simulink model "ReadHectorSlam_Model"  (R2023a)
settings: Solver=FixedStepAuto  StartTime=0.0  StopTime=Inf  RelTol=1e-3
model workspace (MAT data in the model file):
  SL_ROS_VariableLengthArrays_MaxSizes.CommonInfo.ArrayTruncateAction = 'EmitWarning'
  SL_ROS_VariableLengthArrays_MaxSizes.MsgTypeMap = containers.Map
  SL_ROS_VariableLengthArrays_MaxSizes.MsgTypeMap.serialization.keys = {'nav_msgs/OccupancyGrid'}
  SL_ROS_VariableLengthArrays_MaxSizes.MsgTypeMap.serialization.values{1}.PropertyName = 'Data'
  SL_ROS_VariableLengthArrays_MaxSizes.MsgTypeMap.serialization.values{1}.DataType = 'int8'
  SL_ROS_VariableLengthArrays_MaxSizes.MsgTypeMap.serialization.values{1}.MaxLength = 128
  SL_ROS_VariableLengthArrays_MaxSizes.MsgTypeMap.serialization.uniformity = 0
  SL_ROS_VariableLengthArrays_MaxSizes.MsgTypeMap.serialization.keyType = 'char'
  SL_ROS_VariableLengthArrays_MaxSizes.MsgTypeMap.serialization.valueType = 'any'
values from neighbouring files (symbols this model uses):
  map = occupancyMap(cMap,20)    [FrontierPractice.m]    (also in LidarSlam_interp.m = buildMap(scans, poses, obj.mapResolution, obj.maxLidarRange); ReadHectorSlam.m = readOccupancyGrid(mapMsg))
libraries: robotlib x1
settings Model: Creator=cesf9  LastModifiedBy=cesf9
settings OptimizationCC: EnhancedBackFolding=on  PassReuseOutputArgsAs=Individual arguments  ZeroExternalMemoryAtStartup=off  ZeroInternalMemoryAtStartup=off  MaxStackSize=64  OptimizeBlockOrder=speed  DifferentSizesBufferReuse=on  OptimizationCustomize=off  EfficientTunableParamExpr=on
settings DebuggingCC: ParameterTunabilityLossMsg=error
settings HardwareCC: ProdBitPerPointer=32  ProdBitPerSizeT=32  ProdBitPerPtrDiffT=32  ProdLargestAtomicFloat=None  ProdIntDivRoundTo=Undefined  ProdEndianess=Unspecified  ProdWordSize=32  ProdHWDeviceType=Generic->Unspecified (assume 32-bit Generic)  UseEmbeddedCoderFeatures=off
settings SFSimCC: MATLABDynamicMemAlloc=off
settings RTWCC: Description=Embedded Coder  SystemTargetFile=ert.tlc  HardwareBoard=Robot Operating System (ROS)  TLCOptions="-aInlineSetEventsForThisBaseRateFcn=TLC_FALSE -aSuppressMultiTaskScheduler=TLC_FALSE  -aRateBasedStepFcn=0"  TemplateMakefile=ert_default_tmf  Toolchain=Catkin  TargetLang=C++
settings CodeAppCC: ForceParamTrailComments=on  IgnoreCustomStorageClasses=off  OperatorAnnotations=on  SimulinkDataObjDesc=on  SFDataObjDesc=on  InsertBlockDesc=on
settings ERTTargetCC: SupportNonInlinedSFcns=on

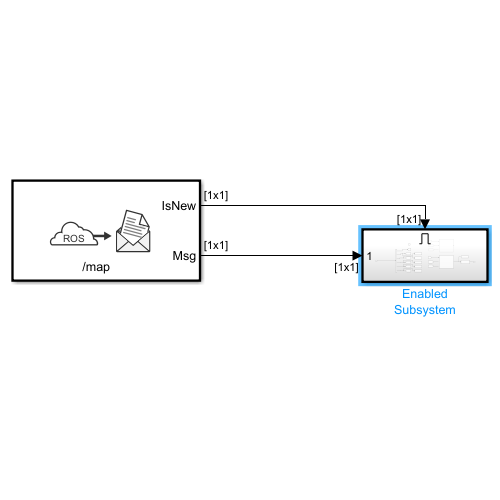
[thumbnail: Simulink's stored preview of the top-level diagram]
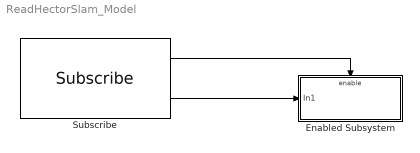
== system ReadHectorSlam_Model ==
  Enabled Subsystem : Subsystem  TreatAsAtomicUnit=on
  Subscribe : robotlib/Subscribe  topicSource=Select from ROS network  topic=/map  messageType=nav_msgs/OccupancyGrid  SampleTime=-1  legacyBusStruct=off  messageQueueLength=1
  wires:
  Subscribe/1 -> Enabled Subsystem/Enable
  Subscribe/2 -> Enabled Subsystem/1(In1)

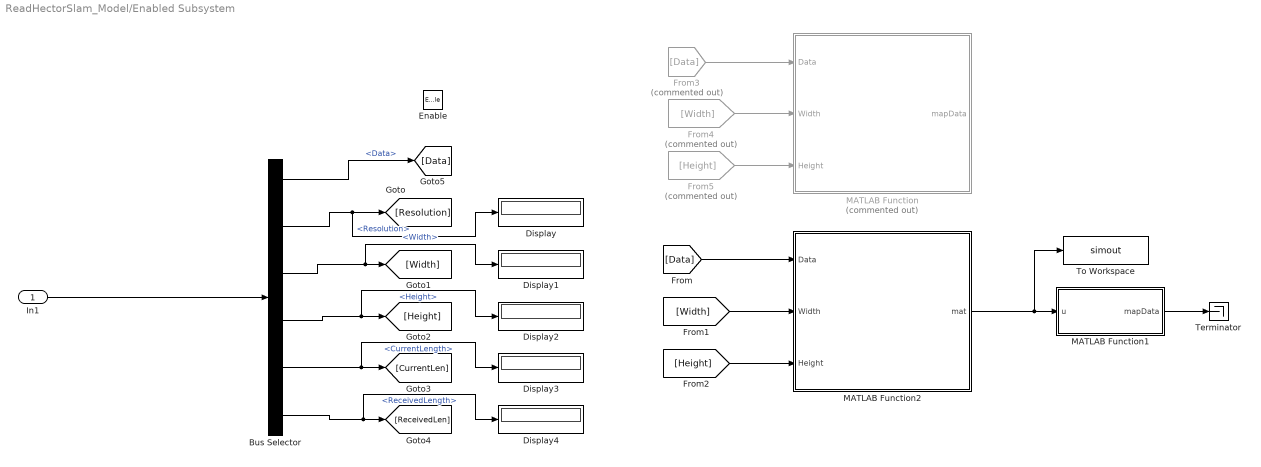
== system ReadHectorSlam_Model/Enabled Subsystem ==
  In1 : Inport
  Enable : EnablePort
  Bus Selector : BusSelector  OutputSignals=Data,Info.Resolution,Info.Width,Info.Height,Data_SL_Info.CurrentLength,Data_SL_Info.ReceivedLength
  Display{,1..4} (5 alike) : Display
  From3 : From  Commented=on  GotoTag=Data
  From4 : From  Commented=on  GotoTag=Width
  From5 : From  Commented=on  GotoTag=Height
  MATLAB Function : MATLAB Function  Commented=on  TreatAsAtomicUnit=on
  MATLAB Function1 : MATLAB Function  TreatAsAtomicUnit=on
  MATLAB Function2 : Subsystem
      mask help: Simulink:masks:GenSFuncDesc_MD
      mask Help: eval('feval(''rtwprivate'',''rtwhelpview'',''rtw_sfcn_block'')');
  Terminator : Terminator
  To Workspace : ToWorkspace  VariableName=simout  SaveFormat=Structure With Time  SampleTime=-1
  wires:
  In1/1 -> Bus Selector/1
  Bus Selector/2 -> Display/1, [Resolution]  "<Resolution>"
  Bus Selector/3 -> Display1/1, [Width]  "<Width>"
  Bus Selector/4 -> Display2/1, [Height]  "<Height>"
  Bus Selector/5 -> Display3/1, [CurrentLen]  "<CurrentLength>"
  Bus Selector/6 -> Display4/1, [ReceivedLen]  "<ReceivedLength>"
  Bus Selector/1 -> [Data]  "<Data>"
  [Data] -> MATLAB Function2/1(Data)
  [Width] -> MATLAB Function2/2(Width)
  [Height] -> MATLAB Function2/3(Height)
  MATLAB Function2/1(mat) -> To Workspace/1, MATLAB Function1/1(u)
  From4/1 -> MATLAB Function/2(Width)
  From3/1 -> MATLAB Function/1(Data)
  From5/1 -> MATLAB Function/3(Height)
  MATLAB Function1/1(mapData) -> Terminator/1

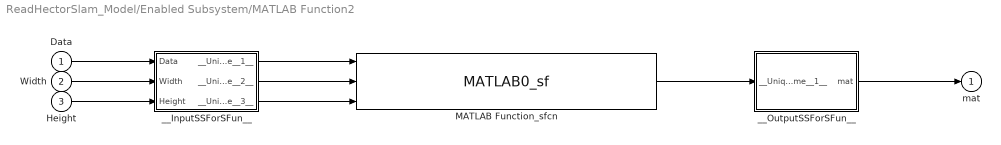
== system ReadHectorSlam_Model/Enabled Subsystem/MATLAB Function2 ==
  Data : Inport
  Width : Inport  Port=2
  Height : Inport  Port=3
  MATLAB Function_sfcn : S-Function  FunctionName=MATLAB0_sf  SFunctionModules=""  SFunctionDeploymentMode=off  EnableBusSupport=off  mask{rtw_sf_name=MATLAB0_sf, showVar=off}
      mask prompts: rtw_sf_name "Simulink:masks:GenSFuncName_MP"; showVar "Simulink:masks:GenSFuncShowModuleList_MP"
      mask help: Simulink:masks:GenSFuncDesc_MD
      mask init:
      | displist = '';
      | if ~strcmp(get_param(gcb, 'FunctionName'), rtw_sf_name);
      |   set_param(gcb, 'FunctionName', rtw_sf_name);
      | end
      | % Check if we are generating code
      | rtw_mode = false;
      | if strcmpi(get_param(bdroot(gcb),'SimulationStatus'),'Initializing')
      | 	rtw_mode = strcmpi(get_param(bdroot(gcb),'BuildingRTWCode'),'on') && ...
      | 		~strcmpi(get_param(bdroot(gcb),'TargetStyle'),'SimulationTarget');
      | end
      | if showVar || rtw_mode
      | 	if exist('rtwsfunc') == 2 | exist('rtwsfunc') == 6
      | 		tmplist = rtwsfunc(rtw_sf_name,gcb);
      | 		tmplist = DAStudio.message('Simulink:masks:GenSFuncListOfModules_IC', tmplist);
      | 	elseif showVar
      | 		tmplist1 = DAStudio.message('Simulink:masks:GenSFuncListOfModules_IC', '');
      |         tmplist2 = DAStudio.message('Simulink:masks:GenSFuncNotLicensed_IC');
      |         tmplist = [tmplist1 tmplist2];
      |  	end
      | end
      | if showVar
      |   displist = tmplist;
      | end
      settings: CopyFcn=|
      | if ~strcmp(get_param(gcb,'Linkstatus'),'none') && ...
      | ~strcmp(get_param(gcb,'Linkstatus'),'implicit')
      |   set_param(gcb,'LinkStatus','none');
      | end
      mask Help: eval('feval(''rtwprivate'',''rtwhelpview'',''rtw_sfcn_block'')');
      mask Display:
      | port_label('input',1,'Data');
      | port_label('input',2,'Width');
      | port_label('input',3,'Height');
      | port_label('output',1,'mat');
  __InputSSForSFun__ : Subsystem
  __OutputSSForSFun__ : Subsystem
  mat : Outport
  wires:
  Data/1 -> __InputSSForSFun__/1(Data)
  Width/1 -> __InputSSForSFun__/2(Width)
  Height/1 -> __InputSSForSFun__/3(Height)
  __InputSSForSFun__/1(__UniqueOutportName__1__) -> MATLAB Function_sfcn/1
  __InputSSForSFun__/2(__UniqueOutportName__2__) -> MATLAB Function_sfcn/2
  __InputSSForSFun__/3(__UniqueOutportName__3__) -> MATLAB Function_sfcn/3
  MATLAB Function_sfcn/1 -> __OutputSSForSFun__/1(__UniqueInportName__1__)
  __OutputSSForSFun__/1(mat) -> mat/1

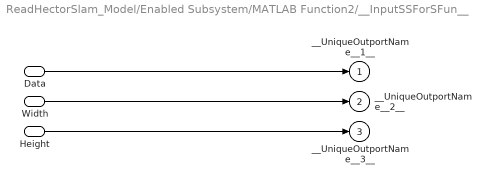
== system ReadHectorSlam_Model/Enabled Subsystem/MATLAB Function2/__InputSSForSFun__ ==
  Data : Inport
  Width : Inport  Port=2
  Height : Inport  Port=3
  __UniqueOutportName__1__ : Outport
  __UniqueOutportName__2__ : Outport  Port=2
  __UniqueOutportName__3__ : Outport  Port=3
  wires:
  Data/1 -> __UniqueOutportName__1__/1
  Width/1 -> __UniqueOutportName__2__/1
  Height/1 -> __UniqueOutportName__3__/1

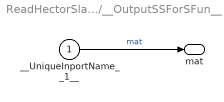
== system ReadHectorSlam_Model/Enabled Subsystem/MATLAB Function2/__OutputSSForSFun__ ==
  __UniqueInportName__1__ : Inport
  mat : Outport
  wires:
  __UniqueInportName__1__/1 -> mat/1  "mat"

== matlab function ReadHectorSlam_Model/Enabled Subsystem/MATLAB Function ==
  data: Data input; mapData output; Width input; Height input
function mapData = msg2matrix(Data,Width,Height)

mapData = zeros(2048,2048,'uint8');

if(Width ~= 0 && Height ~= 0)
    Data(Data < 0) = 50;
    for i = 1:Height
        idxstart = Width*(i-1)+1;
        idxend = Width*i;
        mapData(i,:) = Data(idxstart:idxend);
    end
    mapData = mapData ./ 100;
    
else
    disp("msg2matrix : No Data")
end

== matlab function ReadHectorSlam_Model/Enabled Subsystem/MATLAB Function1 ==
  data: u input; mapData output
function mapData = fcn(u)

if(~isempty(u))
    map = occupancyMap(u,20);
    mapData = occupancyMatrix(map);
    disp(size(mapData))
else
    disp("mapData Fail")
    mapData = zeros(2048,2048);
end
